simulink model "motor_model"  (R2015a)
settings: Solver=ode45  StartTime=0.0  StopTime=10.0  RelTol=1e-3
values from neighbouring files (symbols this model uses):
  Cd = 0.5*1.225*(0.10)^2*1.05    (= 0.00643125)    [Sim.m]
  Cf = 0.9*9.81    (= 8.829)    [Sim.m]
  J = 0.5*mr*Rr^2    (= 3.42e-08)    [Sim.m]
  Kf = 0.26    [Sim.m]    (also in Sim_SS.m = 0.2625)
  Kt = 0.2625    [Sim.m]
  La = 0.05    [Sim.m]
  M = 1    [Sim.m]    (also in Sim_SS.m = 1.5)
  NM = 2    [Sim.m]    (also in Sim_SS.m)
  R = 0.03    [Sim.m]    (also in Sim_SS.m)
  Ra = 5.625    [Sim.m]    (also in Sim_SS.m = 0.0712)
  theta = 5*pi/180    (= 0.0872664625997)    [Sim.m]    (also in Sim_SS.m)
libraries: simulink x1
settings Model: Creator=Paul  LastModifiedBy=miguel

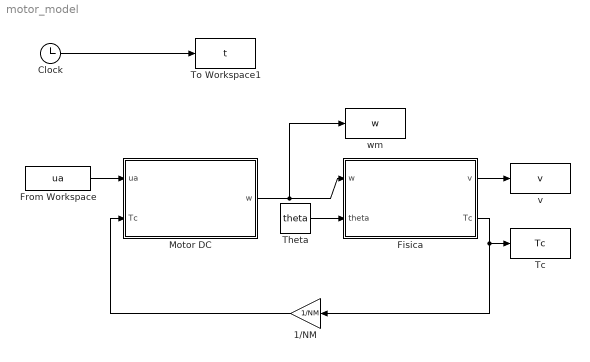
== system motor_model ==
  1/NM : Gain  Gain=1/NM
  Clock : Clock
  Fisica : Subsystem
  From Workspace : FromWorkspace  VariableName=ua  SampleTime=0
  Motor DC : Subsystem
  Tc : ToWorkspace  VariableName=Tc  SampleTime=-1
  Theta : Constant  Value=theta
  To Workspace1 : ToWorkspace  VariableName=t  SampleTime=-1
  v : ToWorkspace  VariableName=v  SampleTime=-1
  wm : ToWorkspace  VariableName=w  SampleTime=-1
  wires:
  Motor DC/1(w) -> wm/1, Fisica/1(w)
  Fisica/1(v) -> v/1
  Fisica/2(Tc) -> Tc/1, 1/NM/1
  1/NM/1 -> Motor DC/2(Tc)
  Theta/1 -> Fisica/2(theta)
  From Workspace/1 -> Motor DC/1("ua ")
  Clock/1 -> To Workspace1/1

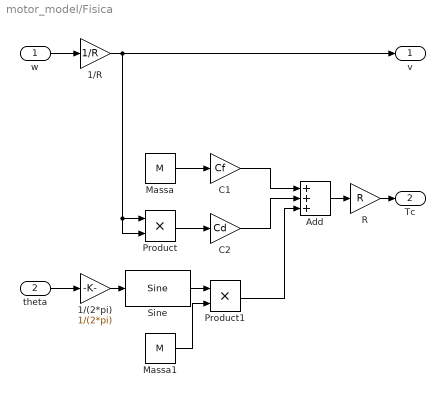
== system motor_model/Fisica ==
  w : Inport
  theta : Inport  Port=2
  1/(2*pi) : Gain  Gain=1/(2*pi)
  1/R : Gain  Gain=1/R
  Add : Sum  Inputs=+++
  C1 : Gain  Gain=Cf
  C2 : Gain  Gain=Cd
  Massa : Constant  Value=M
  Massa1 : Constant  Value=M
  Product : Product
  Product1 : Product
  R : Gain  Gain=R
  Sine : simulink/Lookup Tables/Sine  Formula=sin(2*pi*u)  NumDataPoints=(2^5)+1  OutputWordLength=16  InternalRulePriority=Speed
  v : Outport
  Tc : Outport  Port=2
  wires:
  1/R/1 -> Product/1, Product/2, v/1
  w/1 -> 1/R/1
  R/1 -> Tc/1
  Add/1 -> R/1
  Product/1 -> C2/1
  C2/1 -> Add/2
  Massa/1 -> C1/1
  C1/1 -> Add/1
  Massa1/1 -> Product1/2
  Product1/1 -> Add/3
  Sine/1 -> Product1/1
  1/(2*pi)/1 -> Sine/1
  theta/1 -> 1/(2*pi)/1

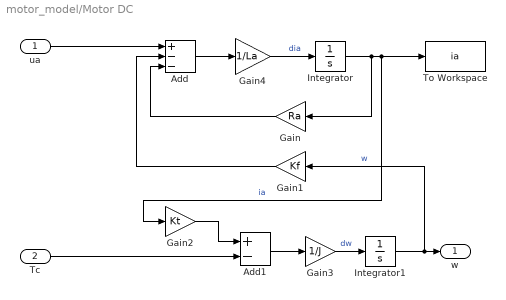
== system motor_model/Motor DC ==
  "ua " : Inport
  Tc : Inport  Port=2
  Add : Sum  Inputs=+--
  Add1 : Sum  Inputs=+-
  Gain : Gain  Gain=Ra
  Gain1 : Gain  Gain=Kf
  Gain2 : Gain  Gain=Kt
  Gain3 : Gain  Gain=1/J
  Gain4 : Gain  Gain=1/La
  Integrator : Integrator
  Integrator1 : Integrator
  To Workspace : ToWorkspace  VariableName=ia  SampleTime=-1
  w : Outport
  wires:
  Integrator/1 -> To Workspace/1, Gain2/1, Gain/1  "ia"
  "ua "/1 -> Add/1
  Add/1 -> Gain4/1
  Gain/1 -> Add/3
  Gain1/1 -> Add/2
  Tc/1 -> Add1/2
  Gain2/1 -> Add1/1
  Integrator1/1 -> w/1, Gain1/1  "w"
  Add1/1 -> Gain3/1
  Gain3/1 -> Integrator1/1  "dw"
  Gain4/1 -> Integrator/1  "dia"
